simulink model "mdaqdemo_can_receive"  (R2014a)
settings: Solver=FixedStepDiscrete  SolverMode=SingleTasking  StartTime=0.0  StopTime=inf  RelTol=1e-3
libraries: microdaq_lib x4, simulink x4
settings Model: SimulationMode=external  CovMetricSettings=dwe  CovHtmlReporting=off  covSaveCumulativeToWorkspaceVar=off  CovSaveSingleToWorkspaceVar=off  CovExternalEMLEnable=on  CovSFcnEnable=on  Creator=skibool  LastModifiedBy=skibool
settings DataIOCC: LimitDataPoints=off  SaveFormat=StructureWithTime
settings OptimizationCC: InlineParams=on  PassReuseOutputArgsAs=Individual arguments  OptimizeModelRefInitCode=on
settings DebuggingCC: MergeDetectMultiDrivingBlocksExec=error  SolverPrmCheckMsg=none  ParameterTunabilityLossMsg=error  FrameProcessingCompatibilityMsg=error  SFUnexpectedBacktrackingDiag=error  SFNoUnconditionalDefaultTransitionDiag=error
settings HardwareCC: ProdBitPerLong=40  ProdLargestAtomicInteger=Integer  ProdIntDivRoundTo=Zero  ProdEndianess=LittleEndian  ProdHWDeviceType=Texas Instruments->C6000
settings ModelReferenceCC: PropagateSignalLabelsOutOfModel=on
settings RTWCC: SystemTargetFile=microdaq.tlc  TemplateMakefile=microdaq.tmf  PostCodeGenCommand=microdaq_postcodegen(buildInfo)  Description=MicroDAQ Real-Time Measurement System  GenerateReport=on  IncludeHyperlinkInReport=on  LaunchReport=on  GenerateTraceInfo=on  GenerateTraceReport=on  GenerateTraceReportSl=on  GenerateTraceReportSf=on  GenerateTraceReportEml=on
settings CodeAppCC: ForceParamTrailComments=on  IgnoreCustomStorageClasses=off  OperatorAnnotations=on  SimulinkDataObjDesc=on  SFDataObjDesc=on  MATLABFcnDesc=on  InsertBlockDesc=on  MATLABSourceComments=on
settings STFCustomTargetCC: TargetLangStandard=C99 (ISO)  MultiwordLength=256  ConcurrentExecutionCompliant=off  GeneratePreprocessorConditionals=Use local settings  CombineOutputUpdateFcns=on  ERTCustomFileBanners=on  SupportContinuousTime=off  SupportNonInlinedSFcns=off  MATLABClassNameForMDSCustomization=Simulink.SoftwareTarget.ERTCustomization  GRTInterface=off  SystemTargetFile=microdaq.tlc
settings ERTTargetCC: TargetLangStandard=C99 (ISO)  MultiwordLength=256  GenerateSampleERTMain=off  ExtMode=on  ExtModeStaticAlloc=on  ExtModeStaticAllocSize=10485760  ExtModeMexArgs=getpref('microdaq','TargetIP') 1 4344  ERTCustomFileTemplate=microdaq_main.tlc  ConvertIfToSwitch=on  SuppressUnreachableDefaultCases=on

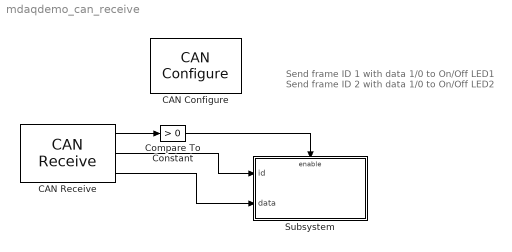
== system mdaqdemo_can_receive ==
  note: Send frame ID 1 with data 1/0 to On/Off LED1
      | Send frame ID 2 with data 1/0 to On/Off LED2
  CAN Configure : microdaq_lib/Network/CAN Configure  SParameter1=500000 kbit/s  SampleTime=-1
  CAN Receive : microdaq_lib/Network/CAN Receive  SampleTime=-1
  Compare To Constant : simulink/Logic and Bit Operations/Compare To Constant  relop=>  const=0  OutDataTypeStr=boolean
  Subsystem : Subsystem
  wires:
  CAN Receive/3 -> Subsystem/2(data)
  Compare To Constant/1 -> Subsystem/Enable
  CAN Receive/1 -> Compare To Constant/1
  CAN Receive/2 -> Subsystem/1(id)

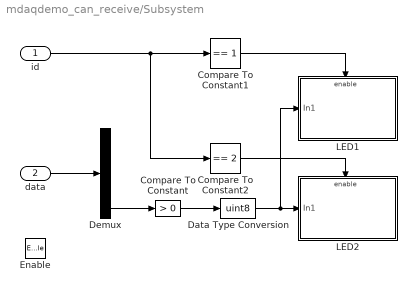
== system mdaqdemo_can_receive/Subsystem ==
  id : Inport
  data : Inport  Port=2
  Enable : EnablePort
  Compare To Constant : simulink/Logic and Bit Operations/Compare To Constant  relop=>  const=0  OutDataTypeStr=boolean
  Compare To Constant1 : simulink/Logic and Bit Operations/Compare To Constant  relop===  const=1  OutDataTypeStr=uint8
  Compare To Constant2 : simulink/Logic and Bit Operations/Compare To Constant  relop===  const=2  OutDataTypeStr=uint8
  Data Type Conversion : DataTypeConversion  OutDataTypeStr=uint8
  Demux : Demux  Outputs=8
  LED1 : Subsystem
  "LED2 " : Subsystem
  wires:
  Compare To Constant1/1 -> LED1/Enable
  Compare To Constant2/1 -> "LED2 "/Enable
  data/1 -> Demux/1
  id/1 -> Compare To Constant2/1, Compare To Constant1/1
  Demux/8 -> Compare To Constant/1
  Data Type Conversion/1 -> LED1/1(In1), "LED2 "/1(In1)
  Compare To Constant/1 -> Data Type Conversion/1

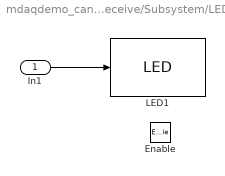
== system mdaqdemo_can_receive/Subsystem/LED1 ==
  In1 : Inport
  Enable : EnablePort
  LED1 : microdaq_lib/Utilities/LED  SParameter1=D1
  wires:
  In1/1 -> LED1/1

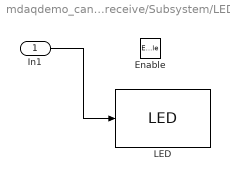
== system mdaqdemo_can_receive/Subsystem/LED2  ==
  In1 : Inport
  Enable : EnablePort
  LED : microdaq_lib/Utilities/LED  SParameter1=D2
  wires:
  In1/1 -> LED/1
